simulink model "buck_converter_data_gen_case1_1"  (R2023b)
settings: Solver=VariableStepAuto  StartTime=0.0  StopTime=Tend  RelTol=1e-3
undefined symbols (not defined in the file or in its folder): Kiv, Kpv, Ts, Tsamp, Ttrig1, Ttrig2, Vg, Vref1, Vref2, Vref3
libraries: spsSeriesRLCBranchLib x3, spsCurrentMeasurementLib x1, spsDCVoltageSourceLib x1, spsDiodeLib x1, spsMosfetLib x1, spsVoltageMeasurementLib x1, simulink_extras x1, spsTriangleGeneratorLib x1, spspowerguiLib x1
settings Model: Creator=baik3-ad  LastModifiedBy=baik3-ad

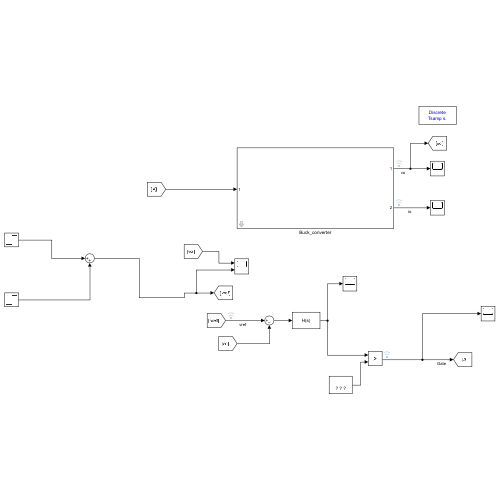
[thumbnail: Simulink's stored preview of the top-level diagram]
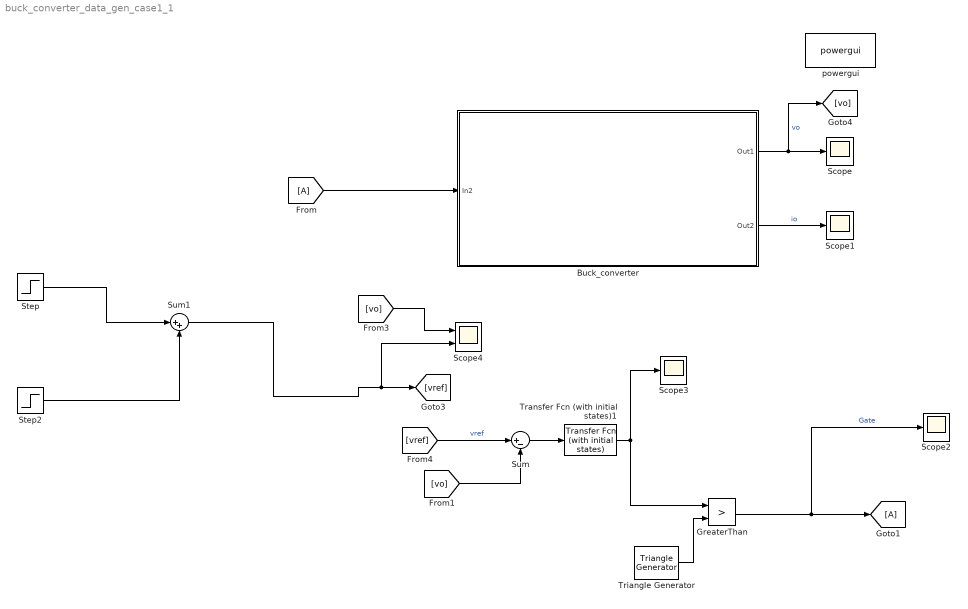
== system buck_converter_data_gen_case1_1 ==
  Buck_converter : Subsystem  mask{Vg=Vg, L=1e-3, C=1e-6, R=10, Rdson=1e-3, Vf=1, Rdon=1e-3}
      mask prompts: Vg "Input voltage"; L "Output inductor"; C "Output capacitor"; R "Output resistor"
  From : From
  Goto1 : Goto
  GreaterThan : RelationalOperator  Operator=>  OutDataTypeStr=fixdt(1,16)  RndMeth=Simplest  InputSameDT=off
  Scope{,1..3} (4 alike) : Scope
  Scope4 : Scope  NumInputPorts=2
  Step : Step  Time=Ttrig1  Before=Vref1  After=Vref2  SampleTime=Tsamp
  Step2 : Step  Time=Ttrig2  After=Vref3-Vref2  SampleTime=Tsamp
  Sum : Sum  Inputs=|+-
  Sum1 : Sum  Inputs=|++
  Transfer Fcn (with initial states)1 : simulink_extras/Additional Linear/Transfer Fcn (with initial states)  N=[Kpv Kiv]  D="[1  0]"  X0=0
  Triangle Generator : spsTriangleGeneratorLib/Triangle Generator  Freq=1/Ts  Phase=0  Ts=Tsamp
  powergui : spspowerguiLib/powergui  Priority=1  SimulationMode=Discrete  SampleTime=Tsamp  frequency=60  Iterations=50  frequencyindice=0  Pbase=100e6  ErrMax=1e-4  UnitsV=kV  UnitsW=MW  buscounter=0  FunctionMessages=off  echomessages=off  EnableUseOfTLC=off  CurrentSourceSwitches=off  DisableSnubberDevices=off  DisableRonSwitches=off  DisableVfSwitches=off  DisplayEquations=off  AutomaticDiscreteSolvers=off  SolverType=Tustin/Backward Euler (TBE)  Interpol=off  ExternalGateDelay=off  methode=off  Ts=100  x0status=blocks  SPID=on  SwTol=0  HookPort=off  NonlinearTolerance=1e-4  nMaxIteration=100  ContinueOnMaxIteration=off  RestoreLinks=warning  ResistiveCurrentMeasurement=off  Frange=[0:2:500]  Ylog=off  Xlog=on  ShowGrid=off  save=off  variable=ZData  structure=0  ZoomFFT=off  StartTime=0.0  cycles=1  DisplayStyle=1  fundamental=60  FreqAxis=off  MaxFrequency=1000  frequencyindicesteady=1  RmsSteady=1  display=off
  wires:
  From/1 -> Buck_converter/1(In2)
  Buck_converter/1(Out1) -> [vo], Scope/1  "vo"
  Buck_converter/2(Out2) -> Scope1/1  "io"
  Sum1/1 -> Scope4/2, [vref]
  GreaterThan/1 -> Scope2/1, Goto1/1  "Gate"
  Sum/1 -> Transfer Fcn (with initial states)1/1
  [vo] -> Sum/2
  Transfer Fcn (with initial states)1/1 -> GreaterThan/1, Scope3/1
  [vref] -> Sum/1  "vref"
  Step/1 -> Sum1/1
  Step2/1 -> Sum1/2
  [vo] -> Scope4/1
  Triangle Generator/1 -> GreaterThan/2

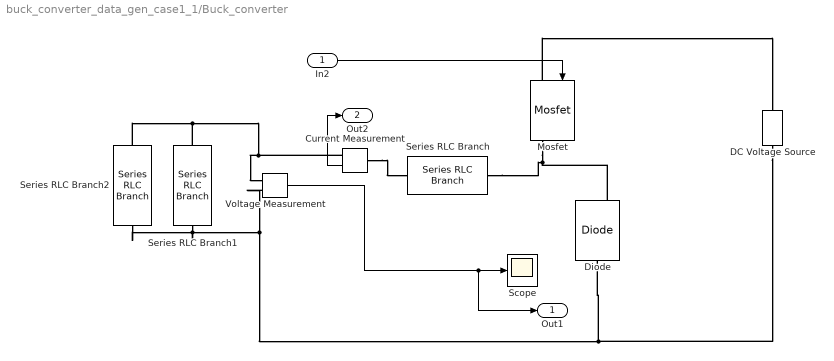
== system buck_converter_data_gen_case1_1/Buck_converter ==
  In2 : Inport
  Current Measurement : spsCurrentMeasurementLib/Current Measurement  PhasorSimulation=off  OutputType=Complex  PSBequivalent=0
  DC Voltage Source : spsDCVoltageSourceLib/DC Voltage Source  Amplitude=Vg  Measurements=None
  Diode : spsDiodeLib/Diode  Ron=Rdon  Lon=0  Vf=Vf  IC=0  UseSnubber=0  Rs=1000  Cs=250e-9  Measurements=on
  Mosfet : spsMosfetLib/Mosfet  Ron=Rdson  Lon=0  Rd=0.01  Vfd=0  IC=0  Rs=1e5  Cs=inf  Measurements=on
  Scope : Scope
  Series RLC Branch : spsSeriesRLCBranchLib/Series RLC Branch  LConnTagsString=__new0  RConnTagsString=__new0  BranchType=L  Resistance=1  Inductance=L  SetiL0=off  InitialCurrent=0  Capacitance=1e-6  Setx0=off  InitialVoltage=0  Measurements=None
  Series RLC Branch1 : spsSeriesRLCBranchLib/Series RLC Branch  LConnTagsString=__new0  RConnTagsString=__new0  BranchType=C  Resistance=1  Inductance=1e-3  SetiL0=off  InitialCurrent=0  Capacitance=C  Setx0=off  InitialVoltage=0  Measurements=None
  Series RLC Branch2 : spsSeriesRLCBranchLib/Series RLC Branch  LConnTagsString=__new0  RConnTagsString=__new0  BranchType=R  Resistance=R  Inductance=1e-3  SetiL0=off  InitialCurrent=0  Capacitance=1e-6  Setx0=off  InitialVoltage=0  Measurements=None
  Voltage Measurement : spsVoltageMeasurementLib/Voltage Measurement  PhasorSimulation=off  OutputType=Complex  PSBequivalent=0
  Out1 : Outport
  Out2 : Outport  Port=2
  wires:
  In2/1 -> Mosfet/1
  Voltage Measurement/1 -> Out1/1, Scope/1
  Current Measurement/1 -> Out2/1
  connections:
  Voltage Measurement/LConn2 -- Series RLC Branch2/RConn1 -- Series RLC Branch1/RConn1 -- DC Voltage Source/LConn1 -- Diode/LConn1
  Series RLC Branch2/LConn1 -- Series RLC Branch1/LConn1 -- Current Measurement/RConn1 -- Voltage Measurement/LConn1
  Mosfet/LConn1 -- DC Voltage Source/RConn1
  Current Measurement/LConn1 -- Series RLC Branch/RConn1
  Series RLC Branch/LConn1 -- Diode/RConn1 -- Mosfet/RConn1
